simulink model "ConSys_A1"  (Simulink 8.3)
settings: Solver=ode3  StartTime=0.0  StopTime=Time(end)  FixedStep=Ts  RelTol=1e-3
values from neighbouring files (symbols this model uses):
  d = r*h    (= 1.6)    [StartUp_A1.m]
  d0 = d*h    (= 0.0032)    [StartUp_A1.m]
  h = 0.002    [StartUp_A1.m]
  Ka = diag([ 3  20  20  150  355  520])    [StartUp_A1.m]
  Kd = diag([ 3   5  25  100   15 1050])    [StartUp_A1.m]
  Ki = diag([35 555 810 7410 1850 5815])    [StartUp_A1.m]
  Kp = diag([55 180 350 1960  680 4450])    [StartUp_A1.m]
  r = 800    [StartUp_A1.m]
  TD = ss(Atd,Btd,Ctd,Dtd,Ts)    [StartUp_A1.m]
  Ts = 1/200    (= 0.005)    [StartUp_A1.m]
undefined symbols (not defined in the file or in its folder): DiscIntNeverNeededParam
undefined symbols (not defined in the file): ADAMS_cwd, ADAMS_exec, ADAMS_host, ADAMS_init, ADAMS_inputs, ADAMS_outputs, ADAMS_prefix, ADAMS_static, ADAMS_sysdir
libraries: cstblocks x6
(part 9 of 9)

== matlab function A2/MATLAB Function 6 ==
  data: q input double; V6 output double; dq input double
function V6 = V6(q,dq)
%#codegen
Th1=q(1,1); Th2=q(2,1); Th3=q(3,1); Th4=q(4,1); Th5=q(5,1); Th6=q(6,1);
dTh1=dq(1); dTh2=dq(2); dTh3=dq(3); dTh4=dq(4); dTh5=dq(5); dTh6=dq(6);
%---------------------------
V611=(0.5*(sin(Th6)*(sin(Th2 + Th3)*sin(Th5) - 1.0*cos(Th2 + Th3)*cos(Th4)*cos(Th5)) - 1.0*cos(Th2 + Th3)*cos(Th6)*sin(Th4))*(0.001043*cos(Th6)*(sin(Th2 + Th3)*sin(Th5) - 1.0*cos(Th2 + Th3)*cos(Th4)*cos(Th5)) - 4.0e-6*sin(Th2 + Th3)*cos(Th5) - 4.0e-6*cos(Th2 + Th3)*cos(Th4)*sin(Th5) + 0.001043*cos(Th2 + Th3)*sin(Th4)*sin(Th6)) - 0.5*(0.00104*cos(Th6)*(sin(Th2 + Th3)*sin(Th5) - 1.0*cos(Th2 + Th3)*cos(Th4)*cos(Th5)) + 0.00104*cos(Th2 + Th3)*sin(Th4)*sin(Th6))*(sin(Th6)*(sin(Th2 + Th3)*sin(Th5) - 1.0*cos(Th2 + Th3)*cos(Th4)*cos(Th5)) - 1.0*cos(Th2 + Th3)*cos(Th6)*sin(Th4)) - 0.5*(sin(Th2 + Th3)*cos(Th5) + cos(Th2 + Th3)*cos(Th4)*sin(Th5))*(4.0e-6*sin(Th6)*(sin(Th2 + Th3)*sin(Th5) - 1.0*cos(Th2 + Th3)*cos(Th4)*cos(Th5)) - 4.0e-6*cos(Th2 + Th3)*cos(Th6)*sin(Th4)) - (0.000115*cos(Th6)*(cos(Th1)*cos(Th4) - 1.0*sin(Th2 + Th3)*sin(Th1)*sin(Th4)) - 0.000115*sin(Th6)*(cos(Th5)*(cos(Th1)*sin(Th4) + sin(Th2 + Th3)*cos(Th4)*sin(Th1)) + cos(Th2 + Th3)*sin(Th1)*sin(Th5)))*(0.07*sin(Th1) + 0.00023*sin(Th6)*(cos(Th1)*cos(Th4) - 1.0*sin(Th2 + Th3)*sin(Th1)*sin(Th4)) + 0.00023*cos(Th6)*(cos(Th5)*(cos(Th1)*sin(Th4) + sin(Th2 + Th3)*cos(Th4)*sin(Th1)) + cos(Th2 + Th3)*sin(Th1)*sin(Th5)) + 0.126*cos(Th2 + Th3)*sin(Th1) - 0.05206*sin(Th5)*(cos(Th1)*sin(Th4) + sin(Th2 + Th3)*cos(Th4)*sin(Th1)) - 0.36*sin(Th1)*sin(Th2) + 0.05206*cos(Th2 + Th3)*cos(Th5)*sin(Th1) + 0.254*cos(Th2)*cos(Th3)*sin(Th1) - 0.254*sin(Th1)*sin(Th2)*sin(Th3)) - 1.0*(0.000115*sin(Th6)*(cos(Th5)*(sin(Th1)*sin(Th4) - 1.0*sin(Th2 + Th3)*cos(Th1)*cos(Th4)) - 1.0*cos(Th2 + Th3)*cos(Th1)*sin(Th5)) - 0.000115*cos(Th6)*(cos(Th4)*sin(Th1) + sin(Th2 + Th3)*cos(Th1)*sin(Th4)))*(0.07*cos(Th1) + 0.05206*sin(Th5)*(sin(Th1)*sin(Th4) - 1.0*sin(Th2 + Th3)*cos(Th1)*cos(Th4)) + 0.126*cos(Th2 + Th3)*cos(Th1) - 0.00023*sin(Th6)*(cos(Th4)*sin(Th1) + sin(Th2 + Th3)*cos(Th1)*sin(Th4)) - 0.36*cos(Th1)*sin(Th2) - 0.00023*cos(Th6)*(cos(Th5)*(sin(Th1)*sin(Th4) - 1.0*sin(Th2 + Th3)*cos(Th1)*cos(Th4)) - 1.0*cos(Th2 + Th3)*cos(Th1)*sin(Th5)) + 0.05206*cos(Th2 + Th3)*cos(Th1)*cos(Th5) + 0.254*cos(Th1)*cos(Th2)*cos(Th3) - 0.254*cos(Th1)*sin(Th2)*sin(Th3)) - 0.5*(0.00104*sin(Th6)*(sin(Th2 + Th3)*sin(Th5) - 1.0*cos(Th2 + Th3)*cos(Th4)*cos(Th5)) - 0.00104*cos(Th2 + Th3)*cos(Th6)*sin(Th4))*(cos(Th6)*(sin(Th2 + Th3)*sin(Th5) - 1.0*cos(Th2 + Th3)*cos(Th4)*cos(Th5)) + cos(Th2 + Th3)*sin(Th4)*sin(Th6)) + 0.5*(0.001043*sin(Th6)*(sin(Th2 + Th3)*sin(Th5) - 1.0*cos(Th2 + Th3)*cos(Th4)*cos(Th5)) - 0.001043*cos(Th2 + Th3)*cos(Th6)*sin(Th4))*(cos(Th6)*(sin(Th2 + Th3)*sin(Th5) - 1.0*cos(Th2 + Th3)*cos(Th4)*cos(Th5)) + cos(Th2 + Th3)*sin(Th4)*sin(Th6)))*dTh1*dTh1;
V612=(0.00011454*cos(Th2)*cos(Th3)*cos(Th5) - 0.0000621*cos(Th2)*cos(Th4)*cos(Th6) - 0.00011454*cos(Th5)*sin(Th2)*sin(Th3) - 0.00006555*cos(Th2)*cos(Th4)*cos(Th6)*sin(Th3) - 0.00006555*cos(Th3)*cos(Th4)*cos(Th6)*sin(Th2) - 4.9934e-6*cos(Th2)*cos(Th3)*cos(Th6)*sin(Th5) - 0.00011751*cos(Th2)*cos(Th4)*sin(Th3)*sin(Th5) - 0.00011751*cos(Th3)*cos(Th4)*sin(Th2)*sin(Th5) + 0.0000621*cos(Th2)*cos(Th5)*sin(Th4)*sin(Th6) + 4.9934e-6*cos(Th2)*sin(Th3)*sin(Th4)*sin(Th6) + 4.9934e-6*cos(Th3)*sin(Th2)*sin(Th4)*sin(Th6) + 4.9934e-6*cos(Th6)*sin(Th2)*sin(Th3)*sin(Th5) + 2.9736e-6*cos(Th2)*cos(Th3)*cos(Th4)^2*cos(Th5) + 2.9736e-6*cos(Th2)*cos(Th3)*cos(Th5)*cos(Th6)^2 - 2.9736e-6*cos(Th4)^2*cos(Th5)*sin(Th2)*sin(Th3) - 2.9736e-6*cos(Th5)*cos(Th6)^2*sin(Th2)*sin(Th3) - 0.00001498*cos(Th2)*cos(Th4)*cos(Th5)*cos(Th6)*sin(Th3) - 0.00001498*cos(Th3)*cos(Th4)*cos(Th5)*cos(Th6)*sin(Th2) + 0.00006555*cos(Th2)*cos(Th5)*sin(Th3)*sin(Th4)*sin(Th6) + 0.00006555*cos(Th3)*cos(Th5)*sin(Th2)*sin(Th4)*sin(Th6) - 9.9869e-6*cos(Th2)*cos(Th3)*cos(Th4)^2*cos(Th6)*sin(Th5) + 2.9736e-6*cos(Th2)*cos(Th4)*cos(Th6)^2*sin(Th3)*sin(Th5) + 2.9736e-6*cos(Th3)*cos(Th4)*cos(Th6)^2*sin(Th2)*sin(Th5) + 9.9869e-6*cos(Th2)*cos(Th5)^2*sin(Th3)*sin(Th4)*sin(Th6) + 9.9869e-6*cos(Th3)*cos(Th5)^2*sin(Th2)*sin(Th4)*sin(Th6) + 9.9869e-6*cos(Th4)^2*cos(Th6)*sin(Th2)*sin(Th3)*sin(Th5) - 5.9471e-6*cos(Th2)*cos(Th3)*cos(Th4)^2*cos(Th5)*cos(Th6)^2 + 5.9471e-6*cos(Th4)^2*cos(Th5)*cos(Th6)^2*sin(Th2)*sin(Th3) + 2.9736e-6*cos(Th2)*cos(Th3)*cos(Th4)*cos(Th6)*sin(Th4)*sin(Th6) - 2.9736e-6*cos(Th4)*cos(Th6)*sin(Th2)*sin(Th3)*sin(Th4)*sin(Th6) - 2.9736e-6*cos(Th4)*cos(Th5)^2*cos(Th6)*sin(Th2)*sin(Th3)*sin(Th4)*sin(Th6) + 9.9869e-6*cos(Th2)*cos(Th3)*cos(Th4)*cos(Th5)*sin(Th4)*sin(Th5)*sin(Th6) - 2.9736e-6*cos(Th2)*cos(Th5)*cos(Th6)*sin(Th3)*sin(Th4)*sin(Th5)*sin(Th6) - 2.9736e-6*cos(Th3)*cos(Th5)*cos(Th6)*sin(Th2)*sin(Th4)*sin(Th5)*sin(Th6) - 9.9869e-6*cos(Th4)*cos(Th5)*sin(Th2)*sin(Th3)*sin(Th4)*sin(Th5)*sin(Th6) + 2.9736e-6*cos(Th2)*cos(Th3)*cos(Th4)*cos(Th5)^2*cos(Th6)*sin(Th4)*sin(Th6))*dTh1*dTh2;
V613=(0.00011454*cos(Th2)*cos(Th3)*cos(Th5) - 0.00011454*cos(Th5)*sin(Th2)*sin(Th3) - 0.00006555*cos(Th2)*cos(Th4)*cos(Th6)*sin(Th3) - 0.00006555*cos(Th3)*cos(Th4)*cos(Th6)*sin(Th2) - 4.9934e-6*cos(Th2)*cos(Th3)*cos(Th6)*sin(Th5) - 0.00011751*cos(Th2)*cos(Th4)*sin(Th3)*sin(Th5) - 0.00011751*cos(Th3)*cos(Th4)*sin(Th2)*sin(Th5) + 4.9934e-6*cos(Th2)*sin(Th3)*sin(Th4)*sin(Th6) + 4.9934e-6*cos(Th3)*sin(Th2)*sin(Th4)*sin(Th6) + 4.9934e-6*cos(Th6)*sin(Th2)*sin(Th3)*sin(Th5) + 2.9736e-6*cos(Th2)*cos(Th3)*cos(Th4)^2*cos(Th5) + 2.9736e-6*cos(Th2)*cos(Th3)*cos(Th5)*cos(Th6)^2 - 2.9736e-6*cos(Th4)^2*cos(Th5)*sin(Th2)*sin(Th3) - 2.9736e-6*cos(Th5)*cos(Th6)^2*sin(Th2)*sin(Th3) - 0.00001498*cos(Th2)*cos(Th4)*cos(Th5)*cos(Th6)*sin(Th3) - 0.00001498*cos(Th3)*cos(Th4)*cos(Th5)*cos(Th6)*sin(Th2) + 0.00006555*cos(Th2)*cos(Th5)*sin(Th3)*sin(Th4)*sin(Th6) + 0.00006555*cos(Th3)*cos(Th5)*sin(Th2)*sin(Th4)*sin(Th6) - 9.9869e-6*cos(Th2)*cos(Th3)*cos(Th4)^2*cos(Th6)*sin(Th5) + 2.9736e-6*cos(Th2)*cos(Th4)*cos(Th6)^2*sin(Th3)*sin(Th5) + 2.9736e-6*cos(Th3)*cos(Th4)*cos(Th6)^2*sin(Th2)*sin(Th5) + 9.9869e-6*cos(Th2)*cos(Th5)^2*sin(Th3)*sin(Th4)*sin(Th6) + 9.9869e-6*cos(Th3)*cos(Th5)^2*sin(Th2)*sin(Th4)*sin(Th6) + 9.9869e-6*cos(Th4)^2*cos(Th6)*sin(Th2)*sin(Th3)*sin(Th5) - 5.9471e-6*cos(Th2)*cos(Th3)*cos(Th4)^2*cos(Th5)*cos(Th6)^2 + 5.9471e-6*cos(Th4)^2*cos(Th5)*cos(Th6)^2*sin(Th2)*sin(Th3) + 2.9736e-6*cos(Th2)*cos(Th3)*cos(Th4)*cos(Th6)*sin(Th4)*sin(Th6) - 2.9736e-6*cos(Th4)*cos(Th6)*sin(Th2)*sin(Th3)*sin(Th4)*sin(Th6) - 2.9736e-6*cos(Th4)*cos(Th5)^2*cos(Th6)*sin(Th2)*sin(Th3)*sin(Th4)*sin(Th6) + 9.9869e-6*cos(Th2)*cos(Th3)*cos(Th4)*cos(Th5)*sin(Th4)*sin(Th5)*sin(Th6) - 2.9736e-6*cos(Th2)*cos(Th5)*cos(Th6)*sin(Th3)*sin(Th4)*sin(Th5)*sin(Th6) - 2.9736e-6*cos(Th3)*cos(Th5)*cos(Th6)*sin(Th2)*sin(Th4)*sin(Th5)*sin(Th6) - 9.9869e-6*cos(Th4)*cos(Th5)*sin(Th2)*sin(Th3)*sin(Th4)*sin(Th5)*sin(Th6) + 2.9736e-6*cos(Th2)*cos(Th3)*cos(Th4)*cos(Th5)^2*cos(Th6)*sin(Th4)*sin(Th6))*dTh1*dTh3;
V614=(0.0000207*cos(Th6)*sin(Th2)*sin(Th4) - 4.025e-6*cos(Th4)*cos(Th5)*sin(Th6) - 4.025e-6*cos(Th6)*sin(Th4) - 0.00001498*cos(Th2)*cos(Th3)*cos(Th4)*sin(Th6) - 0.00002185*cos(Th2)*cos(Th3)*cos(Th6)*sin(Th4) - 0.00011454*cos(Th2)*cos(Th3)*sin(Th4)*sin(Th5) + 2.9736e-6*cos(Th2)*cos(Th6)*sin(Th3)*sin(Th6) + 2.9736e-6*cos(Th3)*cos(Th6)*sin(Th2)*sin(Th6) + 0.0000207*cos(Th4)*cos(Th5)*sin(Th2)*sin(Th6) + 0.00001498*cos(Th4)*sin(Th2)*sin(Th3)*sin(Th6) + 0.00002185*cos(Th6)*sin(Th2)*sin(Th3)*sin(Th4) + 0.00011454*sin(Th2)*sin(Th3)*sin(Th4)*sin(Th5) - 0.00002185*cos(Th2)*cos(Th3)*cos(Th4)*cos(Th5)*sin(Th6) - 4.9934e-6*cos(Th2)*cos(Th3)*cos(Th5)*cos(Th6)*sin(Th4) + 0.00002185*cos(Th4)*cos(Th5)*sin(Th2)*sin(Th3)*sin(Th6) + 4.9934e-6*cos(Th5)*cos(Th6)*sin(Th2)*sin(Th3)*sin(Th4) - 9.9869e-6*cos(Th2)*cos(Th5)*sin(Th3)*sin(Th5)*sin(Th6) - 9.9869e-6*cos(Th3)*cos(Th5)*sin(Th2)*sin(Th5)*sin(Th6) + 9.9869e-6*cos(Th2)*cos(Th3)*cos(Th4)*cos(Th5)^2*sin(Th6) - 2.9736e-6*cos(Th2)*cos(Th3)*cos(Th6)^2*sin(Th4)*sin(Th5) - 2.9736e-6*cos(Th2)*cos(Th5)^2*cos(Th6)*sin(Th3)*sin(Th6) - 2.9736e-6*cos(Th3)*cos(Th5)^2*cos(Th6)*sin(Th2)*sin(Th6) - 9.9869e-6*cos(Th4)*cos(Th5)^2*sin(Th2)*sin(Th3)*sin(Th6) + 2.9736e-6*cos(Th6)^2*sin(Th2)*sin(Th3)*sin(Th4)*sin(Th5) - 2.9736e-6*cos(Th2)*cos(Th3)*cos(Th4)*cos(Th5)*cos(Th6)*sin(Th5)*sin(Th6) + 2.9736e-6*cos(Th4)*cos(Th5)*cos(Th6)*sin(Th2)*sin(Th3)*sin(Th5)*sin(Th6))*dTh1*dTh4;
V615=(4.025e-6*sin(Th4)*sin(Th5)*sin(Th6) - 0.00011751*cos(Th3)*sin(Th2)*sin(Th5) - 0.00011751*cos(Th2)*sin(Th3)*sin(Th5) + 0.00011751*cos(Th2)*cos(Th3)*cos(Th4)*cos(Th5) - 0.00001498*cos(Th2)*cos(Th5)*cos(Th6)*sin(Th3) - 0.00001498*cos(Th3)*cos(Th5)*cos(Th6)*sin(Th2) - 0.00011751*cos(Th4)*cos(Th5)*sin(Th2)*sin(Th3) - 0.0000207*sin(Th2)*sin(Th4)*sin(Th5)*sin(Th6) + 2.9736e-6*cos(Th2)*cos(Th6)^2*sin(Th3)*sin(Th5) + 2.9736e-6*cos(Th3)*cos(Th6)^2*sin(Th2)*sin(Th5) - 0.00001498*cos(Th2)*cos(Th3)*cos(Th4)*cos(Th6)*sin(Th5) + 2.9736e-6*cos(Th2)*cos(Th3)*cos(Th6)*sin(Th4)*sin(Th6) + 0.00002185*cos(Th2)*cos(Th3)*sin(Th4)*sin(Th5)*sin(Th6) + 0.00001498*cos(Th4)*cos(Th6)*sin(Th2)*sin(Th3)*sin(Th5) - 2.9736e-6*cos(Th6)*sin(Th2)*sin(Th3)*sin(Th4)*sin(Th6) - 0.00002185*sin(Th2)*sin(Th3)*sin(Th4)*sin(Th5)*sin(Th6) - 2.9736e-6*cos(Th2)*cos(Th3)*cos(Th4)*cos(Th5)*cos(Th6)^2 + 2.9736e-6*cos(Th4)*cos(Th5)*cos(Th6)^2*sin(Th2)*sin(Th3))*dTh1*dTh5;
V616=(0.0000207*cos(Th4)*sin(Th2)*sin(Th6) - 4.025e-6*cos(Th5)*cos(Th6)*sin(Th4) - 4.025e-6*cos(Th4)*sin(Th6) - 0.00002185*cos(Th2)*cos(Th3)*cos(Th4)*sin(Th6) - 4.9934e-6*cos(Th2)*cos(Th3)*cos(Th6)*sin(Th4) + 0.0000207*cos(Th5)*cos(Th6)*sin(Th2)*sin(Th4) + 0.00002185*cos(Th4)*sin(Th2)*sin(Th3)*sin(Th6) + 4.9934e-6*cos(Th6)*sin(Th2)*sin(Th3)*sin(Th4) + 4.9934e-6*cos(Th2)*sin(Th3)*sin(Th5)*sin(Th6) + 4.9934e-6*cos(Th3)*sin(Th2)*sin(Th5)*sin(Th6) - 4.9934e-6*cos(Th2)*cos(Th3)*cos(Th4)*cos(Th5)*sin(Th6) - 0.00002185*cos(Th2)*cos(Th3)*cos(Th5)*cos(Th6)*sin(Th4) + 4.9934e-6*cos(Th4)*cos(Th5)*sin(Th2)*sin(Th3)*sin(Th6) + 0.00002185*cos(Th5)*cos(Th6)*sin(Th2)*sin(Th3)*sin(Th4))*dTh1*dTh6;
%---------------------------
V621=(2.0e-6*cos(Th2 + Th3)*cos(Th6)*sin(Th5) - 7.245e-6*sin(Th2 + Th3)*cos(Th4)*cos(Th6) - 1.5e-6*cos(Th2 + Th3)*cos(Th5) - 1.5e-6*sin(Th2 + Th3)*cos(Th4)*sin(Th5) - 2.0e-6*sin(Th2 + Th3)*sin(Th4)*sin(Th6) - 0.0000207*cos(Th2)*cos(Th4)*cos(Th6) + 3.0e-6*cos(Th2 + Th3)*cos(Th4)^2*cos(Th5) + 3.0e-6*cos(Th2 + Th3)*cos(Th5)*cos(Th6)^2 - 4.9934e-6*sin(Th2 + Th3)*cos(Th4)*cos(Th5)*cos(Th6) + 7.245e-6*sin(Th2 + Th3)*cos(Th5)*sin(Th4)*sin(Th6) - 0.000014605*cos(Th2)*cos(Th4)*cos(Th6)*sin(Th3) - 0.000014605*cos(Th3)*cos(Th4)*cos(Th6)*sin(Th2) + 0.0000207*cos(Th2)*cos(Th5)*sin(Th4)*sin(Th6) - 6.9935e-6*cos(Th2 + Th3)*cos(Th4)^2*cos(Th6)*sin(Th5) + 2.9935e-6*cos(Th2 + Th3)*cos(Th6)*sin(Th4)^2*sin(Th5) + 2.9868e-6*sin(Th2 + Th3)*cos(Th4)*cos(Th6)^2*sin(Th5) + 1.3225e-8*sin(Th2 + Th3)*cos(Th4)*sin(Th5)*sin(Th6)^2 + 6.9935e-6*sin(Th2 + Th3)*cos(Th5)^2*sin(Th4)*sin(Th6) - 2.9935e-6*sin(Th2 + Th3)*sin(Th4)*sin(Th5)^2*sin(Th6) - 5.9868e-6*cos(Th2 + Th3)*cos(Th4)^2*cos(Th5)*cos(Th6)^2 - 1.3225e-8*cos(Th2 + Th3)*cos(Th5)*cos(Th6)^2*sin(Th4)^2 - 1.3225e-8*cos(Th2 + Th3)*cos(Th4)^2*cos(Th5)*sin(Th6)^2 + 1.3225e-8*cos(Th2 + Th3)*cos(Th5)*sin(Th4)^2*sin(Th6)^2 + 0.000014605*cos(Th2)*cos(Th5)*sin(Th3)*sin(Th4)*sin(Th6) + 0.000014605*cos(Th3)*cos(Th5)*sin(Th2)*sin(Th4)*sin(Th6) + 2.9736e-6*cos(Th2 + Th3)*cos(Th4)*cos(Th6)*sin(Th4)*sin(Th6) + 9.9869e-6*cos(Th2 + Th3)*cos(Th4)*cos(Th5)*sin(Th4)*sin(Th5)*sin(Th6) - 2.9736e-6*sin(Th2 + Th3)*cos(Th5)*cos(Th6)*sin(Th4)*sin(Th5)*sin(Th6) + 2.9736e-6*cos(Th2 + Th3)*cos(Th4)*cos(Th5)^2*cos(Th6)*sin(Th4)*sin(Th6))*dTh2*dTh1;
V622=(0.0000437*sin(Th5)*sin(Th6) - 0.0000414*cos(Th3)*cos(Th6)*sin(Th4) + 2.9736e-6*cos(Th4)*cos(Th5)*sin(Th4) + 9.9869e-6*cos(Th5)*sin(Th5)*sin(Th6) + 0.0000414*sin(Th3)*sin(Th5)*sin(Th6) - 2.9736e-6*cos(Th4)^2*cos(Th6)*sin(Th6) + 2.9736e-6*cos(Th5)^2*cos(Th6)*sin(Th6) - 2.9736e-6*cos(Th4)^2*cos(Th5)^2*cos(Th6)*sin(Th6) - 0.0000414*cos(Th3)*cos(Th4)*cos(Th5)*sin(Th6) - 9.9869e-6*cos(Th4)*cos(Th6)*sin(Th4)*sin(Th5) - 5.9471e-6*cos(Th4)*cos(Th5)*cos(Th6)^2*sin(Th4) - 9.9869e-6*cos(Th4)^2*cos(Th5)*sin(Th5)*sin(Th6))*dTh2*dTh2;
V623=(0.0000437*sin(Th5)*sin(Th6) + 0.0000207*cos(Th3)*cos(Th6)*sin(Th4) + 2.9736e-6*cos(Th4)*cos(Th5)*sin(Th4) + 9.9869e-6*cos(Th5)*sin(Th5)*sin(Th6) - 0.0000207*sin(Th3)*sin(Th5)*sin(Th6) - 2.9736e-6*cos(Th4)^2*cos(Th6)*sin(Th6) + 2.9736e-6*cos(Th5)^2*cos(Th6)*sin(Th6) - 2.9736e-6*cos(Th4)^2*cos(Th5)^2*cos(Th6)*sin(Th6) + 0.0000207*cos(Th3)*cos(Th4)*cos(Th5)*sin(Th6) - 9.9869e-6*cos(Th4)*cos(Th6)*sin(Th4)*sin(Th5) - 5.9471e-6*cos(Th4)*cos(Th5)*cos(Th6)^2*sin(Th4) - 9.9869e-6*cos(Th4)^2*cos(Th5)*sin(Th5)*sin(Th6))*dTh2*dTh3;
V624=(0.00002185*cos(Th4)*cos(Th6) + 0.00011454*cos(Th4)*sin(Th5) - 0.00001498*sin(Th4)*sin(Th6) + 9.9869e-6*cos(Th5)^2*sin(Th4)*sin(Th6) + 4.9934e-6*cos(Th4)*cos(Th5)*cos(Th6) + 0.0000207*cos(Th4)*cos(Th6)*sin(Th3) - 0.00002185*cos(Th5)*sin(Th4)*sin(Th6) + 2.9736e-6*cos(Th4)*cos(Th6)^2*sin(Th5) - 0.0000207*cos(Th5)*sin(Th3)*sin(Th4)*sin(Th6) - 2.9736e-6*cos(Th5)*cos(Th6)*sin(Th4)*sin(Th5)*sin(Th6))*dTh2*dTh4;
V625=(0.00011751*cos(Th5)*sin(Th4) + 0.0000207*cos(Th3)*cos(Th5)*sin(Th6) - 2.9736e-6*cos(Th4)*cos(Th6)*sin(Th6) - 0.00002185*cos(Th4)*sin(Th5)*sin(Th6) - 0.00001498*cos(Th6)*sin(Th4)*sin(Th5) - 2.9736e-6*cos(Th5)*cos(Th6)^2*sin(Th4) - 0.0000207*cos(Th4)*sin(Th3)*sin(Th5)*sin(Th6))*dTh2*dTh5;
V626=(4.9934e-6*cos(Th4)*cos(Th6) - 0.00002185*sin(Th4)*sin(Th6) + 0.00002185*cos(Th4)*cos(Th5)*cos(Th6) + 0.0000207*cos(Th3)*cos(Th6)*sin(Th5) - 4.9934e-6*cos(Th5)*sin(Th4)*sin(Th6) - 0.0000207*sin(Th3)*sin(Th4)*sin(Th6) + 0.0000207*cos(Th4)*cos(Th5)*cos(Th6)*sin(Th3))*dTh2*dTh6;
%---------------------------
V631=(2.0e-6*cos(Th2 + Th3)*cos(Th6)*sin(Th5) - 7.245e-6*sin(Th2 + Th3)*cos(Th4)*cos(Th6) - 1.5e-6*cos(Th2 + Th3)*cos(Th5) - 1.5e-6*sin(Th2 + Th3)*cos(Th4)*sin(Th5) - 2.0e-6*sin(Th2 + Th3)*sin(Th4)*sin(Th6) + 3.0e-6*cos(Th2 + Th3)*cos(Th4)^2*cos(Th5) + 3.0e-6*cos(Th2 + Th3)*cos(Th5)*cos(Th6)^2 - 4.9934e-6*sin(Th2 + Th3)*cos(Th4)*cos(Th5)*cos(Th6) + 7.245e-6*sin(Th2 + Th3)*cos(Th5)*sin(Th4)*sin(Th6) - 0.000014605*cos(Th2)*cos(Th4)*cos(Th6)*sin(Th3) - 0.000014605*cos(Th3)*cos(Th4)*cos(Th6)*sin(Th2) - 6.9935e-6*cos(Th2 + Th3)*cos(Th4)^2*cos(Th6)*sin(Th5) + 2.9935e-6*cos(Th2 + Th3)*cos(Th6)*sin(Th4)^2*sin(Th5) + 2.9868e-6*sin(Th2 + Th3)*cos(Th4)*cos(Th6)^2*sin(Th5) + 1.3225e-8*sin(Th2 + Th3)*cos(Th4)*sin(Th5)*sin(Th6)^2 + 6.9935e-6*sin(Th2 + Th3)*cos(Th5)^2*sin(Th4)*sin(Th6) - 2.9935e-6*sin(Th2 + Th3)*sin(Th4)*sin(Th5)^2*sin(Th6) - 5.9868e-6*cos(Th2 + Th3)*cos(Th4)^2*cos(Th5)*cos(Th6)^2 - 1.3225e-8*cos(Th2 + Th3)*cos(Th5)*cos(Th6)^2*sin(Th4)^2 - 1.3225e-8*cos(Th2 + Th3)*cos(Th4)^2*cos(Th5)*sin(Th6)^2 + 1.3225e-8*cos(Th2 + Th3)*cos(Th5)*sin(Th4)^2*sin(Th6)^2 + 0.000014605*cos(Th2)*cos(Th5)*sin(Th3)*sin(Th4)*sin(Th6) + 0.000014605*cos(Th3)*cos(Th5)*sin(Th2)*sin(Th4)*sin(Th6) + 2.9736e-6*cos(Th2 + Th3)*cos(Th4)*cos(Th6)*sin(Th4)*sin(Th6) + 9.9869e-6*cos(Th2 + Th3)*cos(Th4)*cos(Th5)*sin(Th4)*sin(Th5)*sin(Th6) - 2.9736e-6*sin(Th2 + Th3)*cos(Th5)*cos(Th6)*sin(Th4)*sin(Th5)*sin(Th6) + 2.9736e-6*cos(Th2 + Th3)*cos(Th4)*cos(Th5)^2*cos(Th6)*sin(Th4)*sin(Th6))*dTh3*dTh1;
V632=(0.0000437*sin(Th5)*sin(Th6) - 0.0000207*cos(Th3)*cos(Th6)*sin(Th4) + 2.9736e-6*cos(Th4)*cos(Th5)*sin(Th4) + 9.9869e-6*cos(Th5)*sin(Th5)*sin(Th6) + 0.0000207*sin(Th3)*sin(Th5)*sin(Th6) - 2.9736e-6*cos(Th4)^2*cos(Th6)*sin(Th6) + 2.9736e-6*cos(Th5)^2*cos(Th6)*sin(Th6) - 2.9736e-6*cos(Th4)^2*cos(Th5)^2*cos(Th6)*sin(Th6) - 0.0000207*cos(Th3)*cos(Th4)*cos(Th5)*sin(Th6) - 9.9869e-6*cos(Th4)*cos(Th6)*sin(Th4)*sin(Th5) - 5.9471e-6*cos(Th4)*cos(Th5)*cos(Th6)^2*sin(Th4) - 9.9869e-6*cos(Th4)^2*cos(Th5)*sin(Th5)*sin(Th6))*dTh3*dTh2;
V633=(0.0000437*sin(Th5)*sin(Th6) + 2.9736e-6*cos(Th4)*cos(Th5)*sin(Th4) + 9.9869e-6*cos(Th5)*sin(Th5)*sin(Th6) - 2.9736e-6*cos(Th4)^2*cos(Th6)*sin(Th6) + 2.9736e-6*cos(Th5)^2*cos(Th6)*sin(Th6) - 2.9736e-6*cos(Th4)^2*cos(Th5)^2*cos(Th6)*sin(Th6) - 9.9869e-6*cos(Th4)*cos(Th6)*sin(Th4)*sin(Th5) - 5.9471e-6*cos(Th4)*cos(Th5)*cos(Th6)^2*sin(Th4) - 9.9869e-6*cos(Th4)^2*cos(Th5)*sin(Th5)*sin(Th6))*dTh3*dTh3;
V634=(0.00002185*cos(Th4)*cos(Th6) + 0.00011454*cos(Th4)*sin(Th5) - 0.00001498*sin(Th4)*sin(Th6) + 9.9869e-6*cos(Th5)^2*sin(Th4)*sin(Th6) + 4.9934e-6*cos(Th4)*cos(Th5)*cos(Th6) - 0.00002185*cos(Th5)*sin(Th4)*sin(Th6) + 2.9736e-6*cos(Th4)*cos(Th6)^2*sin(Th5) - 2.9736e-6*cos(Th5)*cos(Th6)*sin(Th4)*sin(Th5)*sin(Th6))*dTh3*dTh4;
V635=(0.00011751*cos(Th5)*sin(Th4) - 2.9736e-6*cos(Th4)*cos(Th6)*sin(Th6) - 0.00002185*cos(Th4)*sin(Th5)*sin(Th6) - 0.00001498*cos(Th6)*sin(Th4)*sin(Th5) - 2.9736e-6*cos(Th5)*cos(Th6)^2*sin(Th4))*dTh3*dTh5;
V636=(4.9934e-6*cos(Th4)*cos(Th6) - 0.00002185*sin(Th4)*sin(Th6) + 0.00002185*cos(Th4)*cos(Th5)*cos(Th6) - 4.9934e-6*cos(Th5)*sin(Th4)*sin(Th6))*dTh3*dTh6;
%---------------------------
V641=(4.025e-6*cos(Th6)*sin(Th4) + 4.025e-6*cos(Th4)*cos(Th5)*sin(Th6) - 0.0000207*cos(Th6)*sin(Th2)*sin(Th4) - 4.9934e-6*cos(Th2)*cos(Th3)*cos(Th4)*sin(Th6) + 0.00002185*cos(Th2)*cos(Th3)*cos(Th6)*sin(Th4) + 1.4868e-6*cos(Th2)*cos(Th3)*sin(Th4)*sin(Th5) + 2.9736e-6*cos(Th2)*cos(Th6)*sin(Th3)*sin(Th6) + 2.9736e-6*cos(Th3)*cos(Th6)*sin(Th2)*sin(Th6) - 0.0000207*cos(Th4)*cos(Th5)*sin(Th2)*sin(Th6) + 4.9934e-6*cos(Th4)*sin(Th2)*sin(Th3)*sin(Th6) - 0.00002185*cos(Th6)*sin(Th2)*sin(Th3)*sin(Th4) - 1.4868e-6*sin(Th2)*sin(Th3)*sin(Th4)*sin(Th5) + 0.00002185*cos(Th2)*cos(Th3)*cos(Th4)*cos(Th5)*sin(Th6) + 4.9934e-6*cos(Th2)*cos(Th3)*cos(Th5)*cos(Th6)*sin(Th4) - 0.00002185*cos(Th4)*cos(Th5)*sin(Th2)*sin(Th3)*sin(Th6) - 4.9934e-6*cos(Th5)*cos(Th6)*sin(Th2)*sin(Th3)*sin(Th4) - 9.9869e-6*cos(Th2)*cos(Th5)*sin(Th3)*sin(Th5)*sin(Th6) - 9.9869e-6*cos(Th3)*cos(Th5)*sin(Th2)*sin(Th5)*sin(Th6) + 9.9869e-6*cos(Th2)*cos(Th3)*cos(Th4)*cos(Th5)^2*sin(Th6) - 2.9736e-6*cos(Th2)*cos(Th3)*cos(Th6)^2*sin(Th4)*sin(Th5) - 2.9736e-6*cos(Th2)*cos(Th5)^2*cos(Th6)*sin(Th3)*sin(Th6) - 2.9736e-6*cos(Th3)*cos(Th5)^2*cos(Th6)*sin(Th2)*sin(Th6) - 9.9869e-6*cos(Th4)*cos(Th5)^2*sin(Th2)*sin(Th3)*sin(Th6) + 2.9736e-6*cos(Th6)^2*sin(Th2)*sin(Th3)*sin(Th4)*sin(Th5) - 2.9736e-6*cos(Th2)*cos(Th3)*cos(Th4)*cos(Th5)*cos(Th6)*sin(Th5)*sin(Th6) + 2.9736e-6*cos(Th4)*cos(Th5)*cos(Th6)*sin(Th2)*sin(Th3)*sin(Th5)*sin(Th6))*dTh4*dTh1;
V642=(9.9869e-6*cos(Th5)^2*sin(Th4)*sin(Th6) - 1.4868e-6*cos(Th4)*sin(Th5) - 4.9934e-6*sin(Th4)*sin(Th6) - 0.00002185*cos(Th4)*cos(Th6) - 4.9934e-6*cos(Th4)*cos(Th5)*cos(Th6) - 0.0000207*cos(Th4)*cos(Th6)*sin(Th3) + 0.00002185*cos(Th5)*sin(Th4)*sin(Th6) + 2.9736e-6*cos(Th4)*cos(Th6)^2*sin(Th5) + 0.0000207*cos(Th5)*sin(Th3)*sin(Th4)*sin(Th6) - 2.9736e-6*cos(Th5)*cos(Th6)*sin(Th4)*sin(Th5)*sin(Th6))*dTh4*dTh2;
V643=(0.00002185*cos(Th5)*sin(Th4)*sin(Th6) - 4.9934e-6*cos(Th4)*cos(Th5)*cos(Th6) - 0.00002185*cos(Th4)*cos(Th6) + 1.4868e-6*cos(Th4)*sin(Th5)*(2.0*cos(Th6)^2 - 1.0) + 4.9934e-6*sin(Th4)*sin(Th6)*(2.0*cos(Th5)^2 - 1.0) - 2.9736e-6*cos(Th5)*cos(Th6)*sin(Th4)*sin(Th5)*sin(Th6))*dTh4*dTh3;
V644=(-8.4703e-27*sin(Th6)*(5.8952e20*sin(2.0*Th5) - 3.5105e20*cos(Th6) + 3.5105e20*cos(Th5)^2*cos(Th6)))*dTh4*dTh4;
V645=(0.5*(0.000115*cos(Th6)*sin(Th1)*sin(Th4) - 0.000115*sin(Th2 + Th3)*cos(Th1)*cos(Th4)*cos(Th6) + 0.000115*cos(Th4)*cos(Th5)*sin(Th1)*sin(Th6) + 0.000115*sin(Th2 + Th3)*cos(Th1)*cos(Th5)*sin(Th4)*sin(Th6))*(0.05206*cos(Th2 + Th3)*cos(Th1)*sin(Th5) - 0.05206*cos(Th5)*sin(Th1)*sin(Th4) + 0.05206*sin(Th2 + Th3)*cos(Th1)*cos(Th4)*cos(Th5) - 0.00023*cos(Th6)*sin(Th1)*sin(Th4)*sin(Th5) - 0.00023*cos(Th2 + Th3)*cos(Th1)*cos(Th5)*cos(Th6) + 0.00023*sin(Th2 + Th3)*cos(Th1)*cos(Th4)*cos(Th6)*sin(Th5)) - 0.0001175*sin(Th5) + 3.0e-6*cos(Th6)^2*sin(Th5) - 6.0e-6*cos(Th5)*cos(Th6) - 0.5*(0.000115*cos(Th1)*cos(Th6)*sin(Th4) + 0.000115*sin(Th2 + Th3)*cos(Th4)*cos(Th6)*sin(Th1) + 0.000115*cos(Th1)*cos(Th4)*cos(Th5)*sin(Th6) - 0.000115*sin(Th2 + Th3)*cos(Th5)*sin(Th1)*sin(Th4)*sin(Th6))*(0.05206*cos(Th2 + Th3)*sin(Th1)*sin(Th5) + 0.05206*cos(Th1)*cos(Th5)*sin(Th4) - 0.00023*cos(Th2 + Th3)*cos(Th5)*cos(Th6)*sin(Th1) + 0.05206*sin(Th2 + Th3)*cos(Th4)*cos(Th5)*sin(Th1) + 0.00023*cos(Th1)*cos(Th6)*sin(Th4)*sin(Th5) + 0.00023*sin(Th2 + Th3)*cos(Th4)*cos(Th6)*sin(Th1)*sin(Th5)) + (0.05206*cos(Th5) + 0.00023*cos(Th6)*sin(Th5))*(0.5*cos(Th1)*cos(Th4) - 0.5*sin(Th2 + Th3)*sin(Th1)*sin(Th4))*(0.00023*sin(Th2 + Th3)*cos(Th6)*sin(Th1)*sin(Th4) - 0.00023*cos(Th1)*cos(Th4)*cos(Th6) + 0.00023*cos(Th2 + Th3)*sin(Th1)*sin(Th5)*sin(Th6) + 0.00023*cos(Th1)*cos(Th5)*sin(Th4)*sin(Th6) + 0.00023*sin(Th2 + Th3)*cos(Th4)*cos(Th5)*sin(Th1)*sin(Th6)) - 0.25*cos(Th2 + Th3)*(0.00023*cos(Th4)*cos(Th6) - 0.00023*cos(Th5)*sin(Th4)*sin(Th6))*(0.05206*cos(Th2 + Th3)*cos(Th4)*cos(Th5) - 0.05206*sin(Th2 + Th3)*sin(Th5) + 0.00023*sin(Th2 + Th3)*cos(Th5)*cos(Th6) + 0.00023*cos(Th2 + Th3)*cos(Th4)*cos(Th6)*sin(Th5)) - 0.0000575*sin(Th6)*(cos(Th2 + Th3)*cos(Th1)*cos(Th5) + sin(Th1)*sin(Th4)*sin(Th5) - 1.0*sin(Th2 + Th3)*cos(Th1)*cos(Th4)*sin(Th5))*(0.05206*cos(Th4)*sin(Th1)*sin(Th5) + 0.00023*sin(Th1)*sin(Th4)*sin(Th6) - 0.00023*sin(Th2 + Th3)*cos(Th1)*cos(Th4)*sin(Th6) + 0.05206*sin(Th2 + Th3)*cos(Th1)*sin(Th4)*sin(Th5) - 0.00023*cos(Th4)*cos(Th5)*cos(Th6)*sin(Th1) - 0.00023*sin(Th2 + Th3)*cos(Th1)*cos(Th5)*cos(Th6)*sin(Th4)) - 0.0000575*sin(Th6)*(cos(Th1)*sin(Th4)*sin(Th5) - 1.0*cos(Th2 + Th3)*cos(Th5)*sin(Th1) + sin(Th2 + Th3)*cos(Th4)*sin(Th1)*sin(Th5))*(0.05206*cos(Th1)*cos(Th4)*sin(Th5) + 0.00023*cos(Th1)*sin(Th4)*sin(Th6) + 0.00023*sin(Th2 + Th3)*cos(Th4)*sin(Th1)*sin(Th6) - 0.05206*sin(Th2 + Th3)*sin(Th1)*sin(Th4)*sin(Th5) - 0.00023*cos(Th1)*cos(Th4)*cos(Th5)*cos(Th6) + 0.00023*sin(Th2 + Th3)*cos(Th5)*cos(Th6)*sin(Th1)*sin(Th4)) - 1.0*(0.05206*cos(Th5) + 0.00023*cos(Th6)*sin(Th5))*(cos(Th4)*sin(Th1) + sin(Th2 + Th3)*cos(Th1)*sin(Th4))*(0.000115*cos(Th4)*cos(Th6)*sin(Th1) + 0.000115*sin(Th2 + Th3)*cos(Th1)*cos(Th6)*sin(Th4) + 0.000115*cos(Th2 + Th3)*cos(Th1)*sin(Th5)*sin(Th6) - 0.000115*cos(Th5)*sin(Th1)*sin(Th4)*sin(Th6) + 0.000115*sin(Th2 + Th3)*cos(Th1)*cos(Th4)*cos(Th5)*sin(Th6)) - 0.0000575*cos(Th2 + Th3)*sin(Th6)*(sin(Th2 + Th3)*cos(Th5) + cos(Th2 + Th3)*cos(Th4)*sin(Th5))*(0.00023*cos(Th4)*sin(Th6) - 0.05206*sin(Th4)*sin(Th5) + 0.00023*cos(Th5)*cos(Th6)*sin(Th4)) - 0.5*cos(Th2 + Th3)*sin(Th4)*(0.05206*cos(Th5) + 0.00023*cos(Th6)*sin(Th5))*(0.00023*cos(Th2 + Th3)*cos(Th6)*sin(Th4) - 0.00023*sin(Th2 + Th3)*sin(Th5)*sin(Th6) + 0.00023*cos(Th2 + Th3)*cos(Th4)*cos(Th5)*sin(Th6)))*dTh4*dTh5;
V646=(0.5*(0.5*(sin(Th5)*(cos(Th1)*sin(Th4) + sin(Th2 + Th3)*cos(Th4)*sin(Th1)) - 1.0*cos(Th2 + Th3)*cos(Th5)*sin(Th1))*(0.00023*sin(Th6)*(sin(Th2 + Th3)*sin(Th5) - 1.0*cos(Th2 + Th3)*cos(Th4)*cos(Th5)) - 0.00023*cos(Th2 + Th3)*cos(Th6)*sin(Th4)) - 0.5*(sin(Th2 + Th3)*cos(Th5) + cos(Th2 + Th3)*cos(Th4)*sin(Th5))*(0.00023*cos(Th6)*(cos(Th1)*cos(Th4) - 1.0*sin(Th2 + Th3)*sin(Th1)*sin(Th4)) - 0.00023*sin(Th6)*(cos(Th5)*(cos(Th1)*sin(Th4) + sin(Th2 + Th3)*cos(Th4)*sin(Th1)) + cos(Th2 + Th3)*sin(Th1)*sin(Th5))))*(0.05206*cos(Th4)*sin(Th1)*sin(Th5) + 0.00023*sin(Th1)*sin(Th4)*sin(Th6) - 0.00023*sin(Th2 + Th3)*cos(Th1)*cos(Th4)*sin(Th6) + 0.05206*sin(Th2 + Th3)*cos(Th1)*sin(Th4)*sin(Th5) - 0.00023*cos(Th4)*cos(Th5)*cos(Th6)*sin(Th1) - 0.00023*sin(Th2 + Th3)*cos(Th1)*cos(Th5)*cos(Th6)*sin(Th4)) - 0.5*(0.5*(sin(Th5)*(sin(Th1)*sin(Th4) - 1.0*sin(Th2 + Th3)*cos(Th1)*cos(Th4)) + cos(Th2 + Th3)*cos(Th1)*cos(Th5))*(0.00023*sin(Th6)*(sin(Th2 + Th3)*sin(Th5) - 1.0*cos(Th2 + Th3)*cos(Th4)*cos(Th5)) - 0.00023*cos(Th2 + Th3)*cos(Th6)*sin(Th4)) + 0.5*(0.00023*sin(Th6)*(cos(Th5)*(sin(Th1)*sin(Th4) - 1.0*sin(Th2 + Th3)*cos(Th1)*cos(Th4)) - 1.0*cos(Th2 + Th3)*cos(Th1)*sin(Th5)) - 0.00023*cos(Th6)*(cos(Th4)*sin(Th1) + sin(Th2 + Th3)*cos(Th1)*sin(Th4)))*(sin(Th2 + Th3)*cos(Th5) + cos(Th2 + Th3)*cos(Th4)*sin(Th5)))*(0.05206*cos(Th1)*cos(Th4)*sin(Th5) + 0.00023*cos(Th1)*sin(Th4)*sin(Th6) + 0.00023*sin(Th2 + Th3)*cos(Th4)*sin(Th1)*sin(Th6) - 0.05206*sin(Th2 + Th3)*sin(Th1)*sin(Th4)*sin(Th5) - 0.00023*cos(Th1)*cos(Th4)*cos(Th5)*cos(Th6) + 0.00023*sin(Th2 + Th3)*cos(Th5)*cos(Th6)*sin(Th1)*sin(Th4)) - 0.5*(0.5*(sin(Th5)*(cos(Th1)*sin(Th4) + sin(Th2 + Th3)*cos(Th4)*sin(Th1)) - 1.0*cos(Th2 + Th3)*cos(Th5)*sin(Th1))*(0.00023*cos(Th6)*(sin(Th2 + Th3)*sin(Th5) - 1.0*cos(Th2 + Th3)*cos(Th4)*cos(Th5)) - 0.01294*sin(Th2 + Th3)*cos(Th5) - 0.01294*cos(Th2 + Th3)*cos(Th4)*sin(Th5) + 0.00023*cos(Th2 + Th3)*sin(Th4)*sin(Th6)) + 0.5*(sin(Th2 + Th3)*cos(Th5) + cos(Th2 + Th3)*cos(Th4)*sin(Th5))*(0.00023*sin(Th6)*(cos(Th1)*cos(Th4) - 1.0*sin(Th2 + Th3)*sin(Th1)*sin(Th4)) + 0.00023*cos(Th6)*(cos(Th5)*(cos(Th1)*sin(Th4) + sin(Th2 + Th3)*cos(Th4)*sin(Th1)) + cos(Th2 + Th3)*sin(Th1)*sin(Th5)) + 0.01294*sin(Th5)*(cos(Th1)*sin(Th4) + sin(Th2 + Th3)*cos(Th4)*sin(Th1)) - 0.01294*cos(Th2 + Th3)*cos(Th5)*sin(Th1)))*(0.00023*cos(Th6)*sin(Th1)*sin(Th4) - 0.00023*sin(Th2 + Th3)*cos(Th1)*cos(Th4)*cos(Th6) + 0.00023*cos(Th4)*cos(Th5)*sin(Th1)*sin(Th6) + 0.00023*sin(Th2 + Th3)*cos(Th1)*cos(Th5)*sin(Th4)*sin(Th6)) + 0.5*(0.5*(sin(Th2 + Th3)*cos(Th5) + cos(Th2 + Th3)*cos(Th4)*sin(Th5))*(0.01294*sin(Th5)*(sin(Th1)*sin(Th4) - 1.0*sin(Th2 + Th3)*cos(Th1)*cos(Th4)) + 0.00023*sin(Th6)*(cos(Th4)*sin(Th1) + sin(Th2 + Th3)*cos(Th1)*sin(Th4)) + 0.00023*cos(Th6)*(cos(Th5)*(sin(Th1)*sin(Th4) - 1.0*sin(Th2 + Th3)*cos(Th1)*cos(Th4)) - 1.0*cos(Th2 + Th3)*cos(Th1)*sin(Th5)) + 0.01294*cos(Th2 + Th3)*cos(Th1)*cos(Th5)) + 0.5*(sin(Th5)*(sin(Th1)*sin(Th4) - 1.0*sin(Th2 + Th3)*cos(Th1)*cos(Th4)) + cos(Th2 + Th3)*cos(Th1)*cos(Th5))*(0.00023*cos(Th6)*(sin(Th2 + Th3)*sin(Th5) - 1.0*cos(Th2 + Th3)*cos(Th4)*cos(Th5)) - 0.01294*sin(Th2 + Th3)*cos(Th5) - 0.01294*cos(Th2 + Th3)*cos(Th4)*sin(Th5) + 0.00023*cos(Th2 + Th3)*sin(Th4)*sin(Th6)))*(0.00023*cos(Th1)*cos(Th6)*sin(Th4) + 0.00023*sin(Th2 + Th3)*cos(Th4)*cos(Th6)*sin(Th1) + 0.00023*cos(Th1)*cos(Th4)*cos(Th5)*sin(Th6) - 0.00023*sin(Th2 + Th3)*cos(Th5)*sin(Th1)*sin(Th4)*sin(Th6)) + 2.0e-6*sin(Th5)*sin(Th6) + 0.25*cos(Th2 + Th3)*(0.00023*cos(Th4)*cos(Th6) - 0.00023*cos(Th5)*sin(Th4)*sin(Th6))*(0.00023*cos(Th2 + Th3)*cos(Th6)*sin(Th4) - 0.00023*sin(Th2 + Th3)*sin(Th5)*sin(Th6) + 0.00023*cos(Th2 + Th3)*cos(Th4)*cos(Th5)*sin(Th6)) - 0.25*cos(Th2 + Th3)*(0.00023*cos(Th4)*sin(Th6) - 0.05206*sin(Th4)*sin(Th5) + 0.00023*cos(Th5)*cos(Th6)*sin(Th4))*(0.00023*cos(Th2 + Th3)*sin(Th4)*sin(Th6) + 0.00023*sin(Th2 + Th3)*cos(Th6)*sin(Th5) - 0.00023*cos(Th2 + Th3)*cos(Th4)*cos(Th5)*cos(Th6)))*dTh4*dTh6;
%---------------------------
V651=(1.4868e-6*cos(Th2)*cos(Th3)*cos(Th4)*cos(Th5) - 1.4868e-6*cos(Th3)*sin(Th2)*sin(Th5) - 4.025e-6*sin(Th4)*sin(Th5)*sin(Th6) - 1.4868e-6*cos(Th2)*sin(Th3)*sin(Th5) - 4.9934e-6*cos(Th2)*cos(Th5)*cos(Th6)*sin(Th3) - 4.9934e-6*cos(Th3)*cos(Th5)*cos(Th6)*sin(Th2) - 1.4868e-6*cos(Th4)*cos(Th5)*sin(Th2)*sin(Th3) + 0.0000207*sin(Th2)*sin(Th4)*sin(Th5)*sin(Th6) + 2.9736e-6*cos(Th2)*cos(Th6)^2*sin(Th3)*sin(Th5) + 2.9736e-6*cos(Th3)*cos(Th6)^2*sin(Th2)*sin(Th5) - 4.9934e-6*cos(Th2)*cos(Th3)*cos(Th4)*cos(Th6)*sin(Th5) + 2.9736e-6*cos(Th2)*cos(Th3)*cos(Th6)*sin(Th4)*sin(Th6) - 0.00002185*cos(Th2)*cos(Th3)*sin(Th4)*sin(Th5)*sin(Th6) + 4.9934e-6*cos(Th4)*cos(Th6)*sin(Th2)*sin(Th3)*sin(Th5) - 2.9736e-6*cos(Th6)*sin(Th2)*sin(Th3)*sin(Th4)*sin(Th6) + 0.00002185*sin(Th2)*sin(Th3)*sin(Th4)*sin(Th5)*sin(Th6) - 2.9736e-6*cos(Th2)*cos(Th3)*cos(Th4)*cos(Th5)*cos(Th6)^2 + 2.9736e-6*cos(Th4)*cos(Th5)*cos(Th6)^2*sin(Th2)*sin(Th3))*dTh5*dTh1;
V652=(1.4868e-6*cos(Th5)*sin(Th4) - 0.0000207*cos(Th3)*cos(Th5)*sin(Th6) - 2.9736e-6*cos(Th4)*cos(Th6)*sin(Th6) + 0.00002185*cos(Th4)*sin(Th5)*sin(Th6) - 4.9934e-6*cos(Th6)*sin(Th4)*sin(Th5) - 2.9736e-6*cos(Th5)*cos(Th6)^2*sin(Th4) + 0.0000207*cos(Th4)*sin(Th3)*sin(Th5)*sin(Th6))*dTh5*dTh2;
V653=(0.00002185*cos(Th4)*sin(Th5)*sin(Th6) - 2.9736e-6*cos(Th4)*cos(Th6)*sin(Th6) - 4.9934e-6*cos(Th6)*sin(Th4)*sin(Th5) - 1.4868e-6*cos(Th5)*sin(Th4)*(2.0*cos(Th6)^2 - 1.0))*dTh5*dTh3;
V654=(3.0e-6*cos(Th6)^2*sin(Th5) - 0.5*(0.000115*cos(Th6)*sin(Th1)*sin(Th4) - 0.000115*sin(Th2 + Th3)*cos(Th1)*cos(Th4)*cos(Th6) + 0.000115*cos(Th4)*cos(Th5)*sin(Th1)*sin(Th6) + 0.000115*sin(Th2 + Th3)*cos(Th1)*cos(Th5)*sin(Th4)*sin(Th6))*(0.05206*cos(Th2 + Th3)*cos(Th1)*sin(Th5) - 0.05206*cos(Th5)*sin(Th1)*sin(Th4) + 0.05206*sin(Th2 + Th3)*cos(Th1)*cos(Th4)*cos(Th5) - 0.00023*cos(Th6)*sin(Th1)*sin(Th4)*sin(Th5) - 0.00023*cos(Th2 + Th3)*cos(Th1)*cos(Th5)*cos(Th6) + 0.00023*sin(Th2 + Th3)*cos(Th1)*cos(Th4)*cos(Th6)*sin(Th5)) - 1.5e-6*sin(Th5) - 2.0e-6*cos(Th5)*cos(Th6) + 0.5*(0.000115*cos(Th1)*cos(Th6)*sin(Th4) + 0.000115*sin(Th2 + Th3)*cos(Th4)*cos(Th6)*sin(Th1) + 0.000115*cos(Th1)*cos(Th4)*cos(Th5)*sin(Th6) - 0.000115*sin(Th2 + Th3)*cos(Th5)*sin(Th1)*sin(Th4)*sin(Th6))*(0.05206*cos(Th2 + Th3)*sin(Th1)*sin(Th5) + 0.05206*cos(Th1)*cos(Th5)*sin(Th4) - 0.00023*cos(Th2 + Th3)*cos(Th5)*cos(Th6)*sin(Th1) + 0.05206*sin(Th2 + Th3)*cos(Th4)*cos(Th5)*sin(Th1) + 0.00023*cos(Th1)*cos(Th6)*sin(Th4)*sin(Th5) + 0.00023*sin(Th2 + Th3)*cos(Th4)*cos(Th6)*sin(Th1)*sin(Th5)) + (0.05206*cos(Th5) + 0.00023*cos(Th6)*sin(Th5))*(0.5*cos(Th1)*cos(Th4) - 0.5*sin(Th2 + Th3)*sin(Th1)*sin(Th4))*(0.00023*sin(Th2 + Th3)*cos(Th6)*sin(Th1)*sin(Th4) - 0.00023*cos(Th1)*cos(Th4)*cos(Th6) + 0.00023*cos(Th2 + Th3)*sin(Th1)*sin(Th5)*sin(Th6) + 0.00023*cos(Th1)*cos(Th5)*sin(Th4)*sin(Th6) + 0.00023*sin(Th2 + Th3)*cos(Th4)*cos(Th5)*sin(Th1)*sin(Th6)) + 0.25*cos(Th2 + Th3)*(0.00023*cos(Th4)*cos(Th6) - 0.00023*cos(Th5)*sin(Th4)*sin(Th6))*(0.05206*cos(Th2 + Th3)*cos(Th4)*cos(Th5) - 0.05206*sin(Th2 + Th3)*sin(Th5) + 0.00023*sin(Th2 + Th3)*cos(Th5)*cos(Th6) + 0.00023*cos(Th2 + Th3)*cos(Th4)*cos(Th6)*sin(Th5)) + 0.0000575*sin(Th6)*(cos(Th2 + Th3)*cos(Th1)*cos(Th5) + sin(Th1)*sin(Th4)*sin(Th5) - 1.0*sin(Th2 + Th3)*cos(Th1)*cos(Th4)*sin(Th5))*(0.05206*cos(Th4)*sin(Th1)*sin(Th5) + 0.00023*sin(Th1)*sin(Th4)*sin(Th6) - 0.00023*sin(Th2 + Th3)*cos(Th1)*cos(Th4)*sin(Th6) + 0.05206*sin(Th2 + Th3)*cos(Th1)*sin(Th4)*sin(Th5) - 0.00023*cos(Th4)*cos(Th5)*cos(Th6)*sin(Th1) - 0.00023*sin(Th2 + Th3)*cos(Th1)*cos(Th5)*cos(Th6)*sin(Th4)) + 0.0000575*sin(Th6)*(cos(Th1)*sin(Th4)*sin(Th5) - 1.0*cos(Th2 + Th3)*cos(Th5)*sin(Th1) + sin(Th2 + Th3)*cos(Th4)*sin(Th1)*sin(Th5))*(0.05206*cos(Th1)*cos(Th4)*sin(Th5) + 0.00023*cos(Th1)*sin(Th4)*sin(Th6) + 0.00023*sin(Th2 + Th3)*cos(Th4)*sin(Th1)*sin(Th6) - 0.05206*sin(Th2 + Th3)*sin(Th1)*sin(Th4)*sin(Th5) - 0.00023*cos(Th1)*cos(Th4)*cos(Th5)*cos(Th6) + 0.00023*sin(Th2 + Th3)*cos(Th5)*cos(Th6)*sin(Th1)*sin(Th4)) - 1.0*(0.05206*cos(Th5) + 0.00023*cos(Th6)*sin(Th5))*(cos(Th4)*sin(Th1) + sin(Th2 + Th3)*cos(Th1)*sin(Th4))*(0.000115*cos(Th4)*cos(Th6)*sin(Th1) + 0.000115*sin(Th2 + Th3)*cos(Th1)*cos(Th6)*sin(Th4) + 0.000115*cos(Th2 + Th3)*cos(Th1)*sin(Th5)*sin(Th6) - 0.000115*cos(Th5)*sin(Th1)*sin(Th4)*sin(Th6) + 0.000115*sin(Th2 + Th3)*cos(Th1)*cos(Th4)*cos(Th5)*sin(Th6)) + 0.0000575*cos(Th2 + Th3)*sin(Th6)*(sin(Th2 + Th3)*cos(Th5) + cos(Th2 + Th3)*cos(Th4)*sin(Th5))*(0.00023*cos(Th4)*sin(Th6) - 0.05206*sin(Th4)*sin(Th5) + 0.00023*cos(Th5)*cos(Th6)*sin(Th4)) - 0.5*cos(Th2 + Th3)*sin(Th4)*(0.05206*cos(Th5) + 0.00023*cos(Th6)*sin(Th5))*(0.00023*cos(Th2 + Th3)*cos(Th6)*sin(Th4) - 0.00023*sin(Th2 + Th3)*sin(Th5)*sin(Th6) + 0.00023*cos(Th2 + Th3)*cos(Th4)*cos(Th5)*sin(Th6)))*dTh5*dTh4;
V655=(-1.4868e-6*sin(2.0*Th6))*dTh5*dTh5;
V656=(4.9934e-6*cos(Th6))*dTh5*dTh6;
%---------------------------
V661=(0)*dTh6*dTh1;
V661=(4.025e-6*cos(Th4)*sin(Th6) + 4.025e-6*cos(Th5)*cos(Th6)*sin(Th4) - 0.0000207*cos(Th4)*sin(Th2)*sin(Th6) + 0.00002185*cos(Th2)*cos(Th3)*cos(Th4)*sin(Th6) + 4.9934e-6*cos(Th2)*cos(Th3)*cos(Th6)*sin(Th4) - 0.0000207*cos(Th5)*cos(Th6)*sin(Th2)*sin(Th4) - 0.00002185*cos(Th4)*sin(Th2)*sin(Th3)*sin(Th6) - 4.9934e-6*cos(Th6)*sin(Th2)*sin(Th3)*sin(Th4) - 4.9934e-6*cos(Th2)*sin(Th3)*sin(Th5)*sin(Th6) - 4.9934e-6*cos(Th3)*sin(Th2)*sin(Th5)*sin(Th6) + 4.9934e-6*cos(Th2)*cos(Th3)*cos(Th4)*cos(Th5)*sin(Th6) + 0.00002185*cos(Th2)*cos(Th3)*cos(Th5)*cos(Th6)*sin(Th4) - 4.9934e-6*cos(Th4)*cos(Th5)*sin(Th2)*sin(Th3)*sin(Th6) - 0.00002185*cos(Th5)*cos(Th6)*sin(Th2)*sin(Th3)*sin(Th4))*dTh6*dTh1;
V662=(0.00002185*sin(Th4)*sin(Th6) - 4.9934e-6*cos(Th4)*cos(Th6) - 0.00002185*cos(Th4)*cos(Th5)*cos(Th6) - 0.0000207*cos(Th3)*cos(Th6)*sin(Th5) + 4.9934e-6*cos(Th5)*sin(Th4)*sin(Th6) + 0.0000207*sin(Th3)*sin(Th4)*sin(Th6) - 0.0000207*cos(Th4)*cos(Th5)*cos(Th6)*sin(Th3))*dTh6*dTh2;
V663=(0.00002185*sin(Th4)*sin(Th6) - 4.9934e-6*cos(Th4)*cos(Th6) - 1.0*(0.00023*cos(Th2 + Th3)*cos(Th6)*sin(Th4) - 0.00023*sin(Th2 + Th3)*sin(Th5)*sin(Th6) + 0.00023*cos(Th2 + Th3)*cos(Th4)*cos(Th5)*sin(Th6))*(0.00023*sin(Th2 + Th3)*cos(Th6)*sin(Th4) + 0.00023*cos(Th2 + Th3)*sin(Th5)*sin(Th6) + 0.00023*sin(Th2 + Th3)*cos(Th4)*cos(Th5)*sin(Th6)) + cos(Th1)*(0.00023*cos(Th2 + Th3)*cos(Th6)*sin(Th4) - 0.00023*sin(Th2 + Th3)*sin(Th5)*sin(Th6) + 0.00023*cos(Th2 + Th3)*cos(Th4)*cos(Th5)*sin(Th6))*(0.00023*cos(Th4)*cos(Th6)*sin(Th1) + 0.00023*sin(Th2 + Th3)*cos(Th1)*cos(Th6)*sin(Th4) + 0.00023*cos(Th2 + Th3)*cos(Th1)*sin(Th5)*sin(Th6) - 0.00023*cos(Th5)*sin(Th1)*sin(Th4)*sin(Th6) + 0.00023*sin(Th2 + Th3)*cos(Th1)*cos(Th4)*cos(Th5)*sin(Th6)) + sin(Th1)*(0.00023*cos(Th2 + Th3)*cos(Th6)*sin(Th4) - 0.00023*sin(Th2 + Th3)*sin(Th5)*sin(Th6) + 0.00023*cos(Th2 + Th3)*cos(Th4)*cos(Th5)*sin(Th6))*(0.00023*sin(Th2 + Th3)*cos(Th6)*sin(Th1)*sin(Th4) - 0.00023*cos(Th1)*cos(Th4)*cos(Th6) + 0.00023*cos(Th2 + Th3)*sin(Th1)*sin(Th5)*sin(Th6) + 0.00023*cos(Th1)*cos(Th5)*sin(Th4)*sin(Th6) + 0.00023*sin(Th2 + Th3)*cos(Th4)*cos(Th5)*sin(Th1)*sin(Th6)) - 0.00002185*cos(Th4)*cos(Th5)*cos(Th6) + 4.9934e-6*cos(Th5)*sin(Th4)*sin(Th6))*dTh6*dTh3;
V664=(0.5*(1.5*(sin(Th2 + Th3)*cos(Th5) + cos(Th2 + Th3)*cos(Th4)*sin(Th5))*(0.00023*sin(Th6)*(cos(Th4)*sin(Th1) + sin(Th2 + Th3)*cos(Th1)*sin(Th4)) - 0.00023*cos(Th6)*(cos(Th2 + Th3)*cos(Th1)*sin(Th5) - 1.0*cos(Th5)*sin(Th1)*sin(Th4) + sin(Th2 + Th3)*cos(Th1)*cos(Th4)*cos(Th5)) + 0.01294*cos(Th2 + Th3)*cos(Th1)*cos(Th5) + 0.01294*sin(Th1)*sin(Th4)*sin(Th5) - 0.01294*sin(Th2 + Th3)*cos(Th1)*cos(Th4)*sin(Th5)) - 1.5*(cos(Th2 + Th3)*cos(Th1)*cos(Th5) + sin(Th1)*sin(Th4)*sin(Th5) - 1.0*sin(Th2 + Th3)*cos(Th1)*cos(Th4)*sin(Th5))*(0.01294*sin(Th2 + Th3)*cos(Th5) + 0.01294*cos(Th2 + Th3)*cos(Th4)*sin(Th5) - 0.00023*cos(Th2 + Th3)*sin(Th4)*sin(Th6) - 0.00023*sin(Th2 + Th3)*cos(Th6)*sin(Th5) + 0.00023*cos(Th2 + Th3)*cos(Th4)*cos(Th5)*cos(Th6)))*(0.00023*cos(Th1)*cos(Th6)*sin(Th4) + 0.00023*sin(Th2 + Th3)*cos(Th4)*cos(Th6)*sin(Th1) + 0.00023*cos(Th1)*cos(Th4)*cos(Th5)*sin(Th6) - 0.00023*sin(Th2 + Th3)*cos(Th5)*sin(Th1)*sin(Th4)*sin(Th6)) - 0.5*(0.5*(cos(Th2 + Th3)*cos(Th1)*cos(Th5) + sin(Th1)*sin(Th4)*sin(Th5) - 1.0*sin(Th2 + Th3)*cos(Th1)*cos(Th4)*sin(Th5))*(0.00023*cos(Th2 + Th3)*cos(Th6)*sin(Th4) - 0.00023*sin(Th2 + Th3)*sin(Th5)*sin(Th6) + 0.00023*cos(Th2 + Th3)*cos(Th4)*cos(Th5)*sin(Th6)) + 0.5*(0.00023*sin(Th6)*(cos(Th2 + Th3)*cos(Th1)*sin(Th5) - 1.0*cos(Th5)*sin(Th1)*sin(Th4) + sin(Th2 + Th3)*cos(Th1)*cos(Th4)*cos(Th5)) + 0.00023*cos(Th6)*(cos(Th4)*sin(Th1) + sin(Th2 + Th3)*cos(Th1)*sin(Th4)))*(sin(Th2 + Th3)*cos(Th5) + cos(Th2 + Th3)*cos(Th4)*sin(Th5)))*(0.05206*cos(Th1)*cos(Th4)*sin(Th5) + 0.00023*cos(Th1)*sin(Th4)*sin(Th6) + 0.00023*sin(Th2 + Th3)*cos(Th4)*sin(Th1)*sin(Th6) - 0.05206*sin(Th2 + Th3)*sin(Th1)*sin(Th4)*sin(Th5) - 0.00023*cos(Th1)*cos(Th4)*cos(Th5)*cos(Th6) + 0.00023*sin(Th2 + Th3)*cos(Th5)*cos(Th6)*sin(Th1)*sin(Th4)) - 0.5*(1.5*(sin(Th2 + Th3)*cos(Th5) + cos(Th2 + Th3)*cos(Th4)*sin(Th5))*(0.00023*cos(Th6)*(cos(Th2 + Th3)*sin(Th1)*sin(Th5) + cos(Th1)*cos(Th5)*sin(Th4) + sin(Th2 + Th3)*cos(Th4)*cos(Th5)*sin(Th1)) + 0.00023*sin(Th6)*(cos(Th1)*cos(Th4) - 1.0*sin(Th2 + Th3)*sin(Th1)*sin(Th4)) - 0.01294*cos(Th2 + Th3)*cos(Th5)*sin(Th1) + 0.01294*cos(Th1)*sin(Th4)*sin(Th5) + 0.01294*sin(Th2 + Th3)*cos(Th4)*sin(Th1)*sin(Th5)) - 1.5*(cos(Th1)*sin(Th4)*sin(Th5) - 1.0*cos(Th2 + Th3)*cos(Th5)*sin(Th1) + sin(Th2 + Th3)*cos(Th4)*sin(Th1)*sin(Th5))*(0.01294*sin(Th2 + Th3)*cos(Th5) + 0.01294*cos(Th2 + Th3)*cos(Th4)*sin(Th5) - 0.00023*cos(Th2 + Th3)*sin(Th4)*sin(Th6) - 0.00023*sin(Th2 + Th3)*cos(Th6)*sin(Th5) + 0.00023*cos(Th2 + Th3)*cos(Th4)*cos(Th5)*cos(Th6)))*(0.00023*cos(Th6)*sin(Th1)*sin(Th4) - 0.00023*sin(Th2 + Th3)*cos(Th1)*cos(Th4)*cos(Th6) + 0.00023*cos(Th4)*cos(Th5)*sin(Th1)*sin(Th6) + 0.00023*sin(Th2 + Th3)*cos(Th1)*cos(Th5)*sin(Th4)*sin(Th6)) + 0.5*(0.5*(cos(Th1)*sin(Th4)*sin(Th5) - 1.0*cos(Th2 + Th3)*cos(Th5)*sin(Th1) + sin(Th2 + Th3)*cos(Th4)*sin(Th1)*sin(Th5))*(0.00023*cos(Th2 + Th3)*cos(Th6)*sin(Th4) - 0.00023*sin(Th2 + Th3)*sin(Th5)*sin(Th6) + 0.00023*cos(Th2 + Th3)*cos(Th4)*cos(Th5)*sin(Th6)) + 0.5*(sin(Th2 + Th3)*cos(Th5) + cos(Th2 + Th3)*cos(Th4)*sin(Th5))*(0.00023*cos(Th6)*(cos(Th1)*cos(Th4) - 1.0*sin(Th2 + Th3)*sin(Th1)*sin(Th4)) - 0.00023*sin(Th6)*(cos(Th2 + Th3)*sin(Th1)*sin(Th5) + cos(Th1)*cos(Th5)*sin(Th4) + sin(Th2 + Th3)*cos(Th4)*cos(Th5)*sin(Th1))))*(0.05206*cos(Th4)*sin(Th1)*sin(Th5) + 0.00023*sin(Th1)*sin(Th4)*sin(Th6) - 0.00023*sin(Th2 + Th3)*cos(Th1)*cos(Th4)*sin(Th6) + 0.05206*sin(Th2 + Th3)*cos(Th1)*sin(Th4)*sin(Th5) - 0.00023*cos(Th4)*cos(Th5)*cos(Th6)*sin(Th1) - 0.00023*sin(Th2 + Th3)*cos(Th1)*cos(Th5)*cos(Th6)*sin(Th4)) - 2.0e-6*sin(Th5)*sin(Th6) + 0.75*cos(Th2 + Th3)*(0.00023*cos(Th4)*cos(Th6) - 0.00023*cos(Th5)*sin(Th4)*sin(Th6))*(0.00023*cos(Th2 + Th3)*cos(Th6)*sin(Th4) - 0.00023*sin(Th2 + Th3)*sin(Th5)*sin(Th6) + 0.00023*cos(Th2 + Th3)*cos(Th4)*cos(Th5)*sin(Th6)) + 0.25*cos(Th2 + Th3)*(0.00023*cos(Th4)*sin(Th6) - 0.05206*sin(Th4)*sin(Th5) + 0.00023*cos(Th5)*cos(Th6)*sin(Th4))*(0.00023*cos(Th2 + Th3)*sin(Th4)*sin(Th6) + 0.00023*sin(Th2 + Th3)*cos(Th6)*sin(Th5) - 0.00023*cos(Th2 + Th3)*cos(Th4)*cos(Th5)*cos(Th6)))*dTh6*dTh4;
V665=(0.5*(0.000115*cos(Th2 + Th3)*sin(Th4)*sin(Th6) + 0.000115*sin(Th2 + Th3)*cos(Th6)*sin(Th5) - 0.000115*cos(Th2 + Th3)*cos(Th4)*cos(Th5)*cos(Th6))*(0.05206*cos(Th2 + Th3)*cos(Th4)*cos(Th5) - 0.05206*sin(Th2 + Th3)*sin(Th5) + 0.00023*sin(Th2 + Th3)*cos(Th5)*cos(Th6) + 0.00023*cos(Th2 + Th3)*cos(Th4)*cos(Th6)*sin(Th5)) - 2.0e-6*cos(Th6) - 0.5*(0.5*(cos(Th2 + Th3)*cos(Th1)*cos(Th5) + sin(Th1)*sin(Th4)*sin(Th5) - 1.0*sin(Th2 + Th3)*cos(Th1)*cos(Th4)*sin(Th5))*(0.00023*cos(Th2 + Th3)*cos(Th6)*sin(Th4) - 0.00023*sin(Th2 + Th3)*sin(Th5)*sin(Th6) + 0.00023*cos(Th2 + Th3)*cos(Th4)*cos(Th5)*sin(Th6)) + 0.5*(0.00023*sin(Th6)*(cos(Th2 + Th3)*cos(Th1)*sin(Th5) - 1.0*cos(Th5)*sin(Th1)*sin(Th4) + sin(Th2 + Th3)*cos(Th1)*cos(Th4)*cos(Th5)) + 0.00023*cos(Th6)*(cos(Th4)*sin(Th1) + sin(Th2 + Th3)*cos(Th1)*sin(Th4)))*(sin(Th2 + Th3)*cos(Th5) + cos(Th2 + Th3)*cos(Th4)*sin(Th5)))*(0.05206*cos(Th2 + Th3)*sin(Th1)*sin(Th5) + 0.05206*cos(Th1)*cos(Th5)*sin(Th4) - 0.00023*cos(Th2 + Th3)*cos(Th5)*cos(Th6)*sin(Th1) + 0.05206*sin(Th2 + Th3)*cos(Th4)*cos(Th5)*sin(Th1) + 0.00023*cos(Th1)*cos(Th6)*sin(Th4)*sin(Th5) + 0.00023*sin(Th2 + Th3)*cos(Th4)*cos(Th6)*sin(Th1)*sin(Th5)) - 0.5*(0.5*(cos(Th1)*sin(Th4)*sin(Th5) - 1.0*cos(Th2 + Th3)*cos(Th5)*sin(Th1) + sin(Th2 + Th3)*cos(Th4)*sin(Th1)*sin(Th5))*(0.00023*cos(Th2 + Th3)*cos(Th6)*sin(Th4) - 0.00023*sin(Th2 + Th3)*sin(Th5)*sin(Th6) + 0.00023*cos(Th2 + Th3)*cos(Th4)*cos(Th5)*sin(Th6)) + 0.5*(sin(Th2 + Th3)*cos(Th5) + cos(Th2 + Th3)*cos(Th4)*sin(Th5))*(0.00023*cos(Th6)*(cos(Th1)*cos(Th4) - 1.0*sin(Th2 + Th3)*sin(Th1)*sin(Th4)) - 0.00023*sin(Th6)*(cos(Th2 + Th3)*sin(Th1)*sin(Th5) + cos(Th1)*cos(Th5)*sin(Th4) + sin(Th2 + Th3)*cos(Th4)*cos(Th5)*sin(Th1))))*(0.05206*cos(Th2 + Th3)*cos(Th1)*sin(Th5) - 0.05206*cos(Th5)*sin(Th1)*sin(Th4) + 0.05206*sin(Th2 + Th3)*cos(Th1)*cos(Th4)*cos(Th5) - 0.00023*cos(Th6)*sin(Th1)*sin(Th4)*sin(Th5) - 0.00023*cos(Th2 + Th3)*cos(Th1)*cos(Th5)*cos(Th6) + 0.00023*sin(Th2 + Th3)*cos(Th1)*cos(Th4)*cos(Th6)*sin(Th5)) + 0.0001725*sin(Th6)*(cos(Th2 + Th3)*cos(Th1)*cos(Th5) + sin(Th1)*sin(Th4)*sin(Th5) - 1.0*sin(Th2 + Th3)*cos(Th1)*cos(Th4)*sin(Th5))*(0.00023*cos(Th4)*cos(Th6)*sin(Th1) + 0.00023*sin(Th2 + Th3)*cos(Th1)*cos(Th6)*sin(Th4) + 0.00023*cos(Th2 + Th3)*cos(Th1)*sin(Th5)*sin(Th6) - 0.00023*cos(Th5)*sin(Th1)*sin(Th4)*sin(Th6) + 0.00023*sin(Th2 + Th3)*cos(Th1)*cos(Th4)*cos(Th5)*sin(Th6)) - 0.0001725*sin(Th6)*(cos(Th1)*sin(Th4)*sin(Th5) - 1.0*cos(Th2 + Th3)*cos(Th5)*sin(Th1) + sin(Th2 + Th3)*cos(Th4)*sin(Th1)*sin(Th5))*(0.00023*sin(Th2 + Th3)*cos(Th6)*sin(Th1)*sin(Th4) - 0.00023*cos(Th1)*cos(Th4)*cos(Th6) + 0.00023*cos(Th2 + Th3)*sin(Th1)*sin(Th5)*sin(Th6) + 0.00023*cos(Th1)*cos(Th5)*sin(Th4)*sin(Th6) + 0.00023*sin(Th2 + Th3)*cos(Th4)*cos(Th5)*sin(Th1)*sin(Th6)) - 0.000115*sin(Th6)*(1.5*sin(Th2 + Th3)*cos(Th5) + 1.5*cos(Th2 + Th3)*cos(Th4)*sin(Th5))*(0.00023*cos(Th2 + Th3)*cos(Th6)*sin(Th4) - 0.00023*sin(Th2 + Th3)*sin(Th5)*sin(Th6) + 0.00023*cos(Th2 + Th3)*cos(Th4)*cos(Th5)*sin(Th6)))*dTh6*dTh5;
V666=(0)*dTh6*dTh6;
%---------------------------
V6 = V611+V612+V613+V614+V615+V616+V621+V622+V623+V624+V625+V626+...
     V631+V632+V633+V634+V635+V636+V641+V642+V643+V644+V645+V646+...
     V651+V652+V653+V654+V655+V656+V661+V662+V663+V664+V665+V666;
end
